simulink model "ex_2_1_si"  (R2022b)
settings: Solver=VariableStepAuto  StartTime=0.0  StopTime=T_sim  RelTol=1e-3
values from neighbouring files (symbols this model uses):
  A = pi*r^2    (= 0.00220618344098)    [ex_2_1_constantes.m]
  A0 = pi*(d/2)^2    (= 4.90873852123e-06)    [ex_2_1_constantes.m]
  C = 0.22e-6    (= 2.2e-07)    [ex_2_1_constantes.m]
  R = 250e6    (= 250000000)    [ex_2_1_constantes.m]
  V_0 = A*L    (= 0.0020296887657)    [ex_2_1_constantes.m]
settings Model: Creator=nicol  LastModifiedBy=nicol

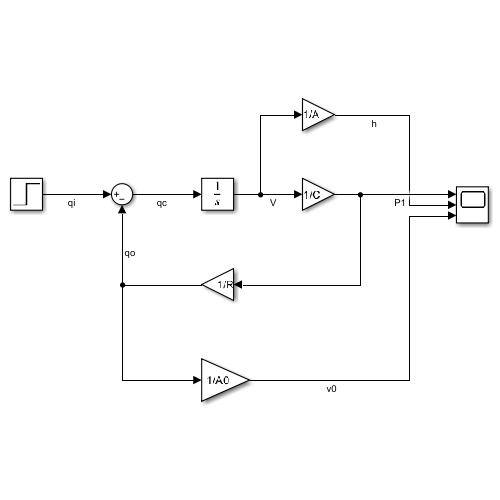
[thumbnail: Simulink's stored preview of the top-level diagram]
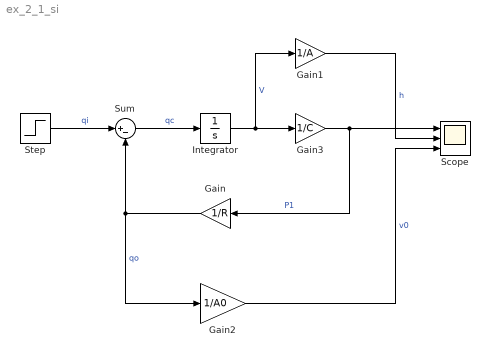
== system ex_2_1_si ==
  Gain : Gain  Gain=1/R
  Gain1 : Gain  Gain=1/A
  Gain2 : Gain  Gain=1/A0
  Gain3 : Gain  Gain=1/C
  Integrator : Integrator  InitialCondition=V_0
  Scope : Scope  NumInputPorts=3
  Step : Step  Time=0  After=0  SampleTime=0
  Sum : Sum  Inputs=|+-
  wires:
  Step/1 -> Sum/1  "qi"
  Sum/1 -> Integrator/1  "qc"
  Integrator/1 -> Gain1/1, Gain3/1  "V"
  Gain3/1 -> Scope/1, Gain/1  "P1"
  Gain1/1 -> Scope/2  "h"
  Gain/1 -> Gain2/1, Sum/2  "qo"
  Gain2/1 -> Scope/3  "v0"
